simulink model "energy_storage_dclink"  (R2018a)
settings: Solver=ode4  StartTime=0.0  StopTime=sim.tTotal  FixedStep=sim.tStep  RelTol=1e-3
undefined symbols (not defined in the file or in its folder): D11, Delta, grid, sim, Vbase, vsc
libraries: powerlib x12, pwrsys x12
settings Model: Creator=ericfa  LastModifiedBy=ericfa

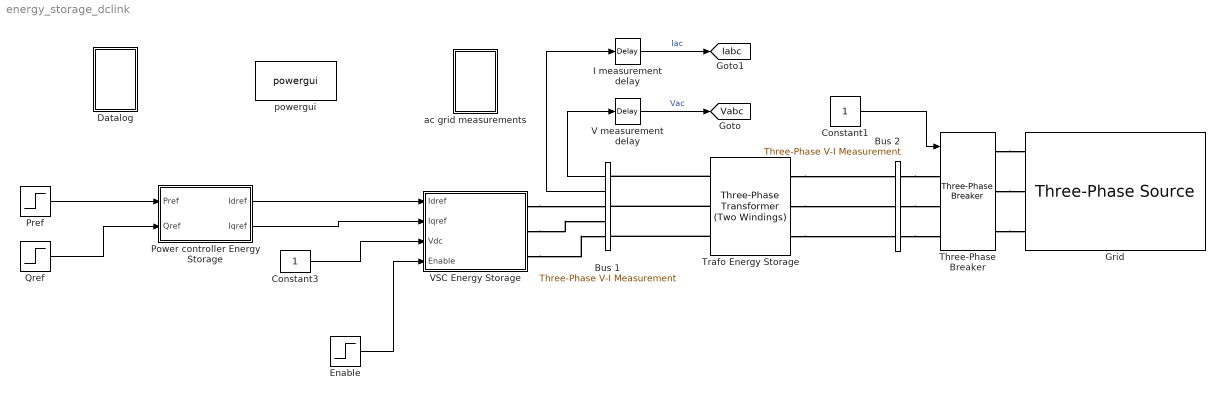
== system energy_storage_dclink ==
  Bus 1 : powerlib/Measurements/Three-Phase V-I Measurement  VoltageMeasurement=phase-to-ground  SetLabelV=off  LabelV=Vabc  Vpu=off  VpuLL=off  CurrentMeasurement=yes  SetLabelI=off  LabelI=Iabc  Ipu=off  Pbase=Sbase  Vbase=Vbase*sqrt(3/2)  OutputType=Complex  PhasorSimulation=off  PSBequivalent=0
  Bus 2 : powerlib/Measurements/Three-Phase V-I Measurement  VoltageMeasurement=phase-to-ground  SetLabelV=on  LabelV=Vabc_B2  Vpu=off  VpuLL=off  CurrentMeasurement=yes  SetLabelI=on  LabelI=Iabc_B2  Ipu=off  Pbase=100e6  Vbase=500e3  OutputType=Magnitude  PhasorSimulation=off  PSBequivalent=0
      settings: SourceProductName=Simscape Electrical
  Constant1 : Constant
  Constant3 : Constant
  Datalog : Subsystem
  Enable : Step  Time=0.05  SampleTime=0
  Grid : powerlib/Electrical Sources/Three-Phase Source  InternalConnection=Yg  VoltagePhases=off  Voltage=grid.UB2  PhaseAngle=0  Voltage_phases=[25e3 25e3 25e3]/sqrt(3)  PhaseAngles_phases=[0 -120 +120]  Frequency=grid.fn  NonIdealSource=on  SpecifyImpedance=on  Resistance=0.8929  Inductance=16.58e-3  ShortCircuitLevel=10*vsc.Sbase  BaseVoltage=grid.UB2  XRratio=10  BusType=swing  Pref=0  Qref=0  Prefabc=[10e3, 10e3, 10e3]  Qrefabc=[0, 0, 0]  Qmin=-inf  Qmax=inf
      settings: SourceProductName=Simscape Electrical
  I measurement delay : TransportDelay  DelayTime=sim.tStep; % 1/vsc.fSwitch
  Power controller Energy Storage : Subsystem
  Pref : Step  Time=0.4  After=0.5  SampleTime=0
  Qref : Step  Time=0.7  After=0.5  SampleTime=0
  Three-Phase Breaker : powerlib/Elements/Three-Phase Breaker  InitialState=open  SwitchA=on  SwitchB=on  SwitchC=on  SwitchTimes="[1/60  5/60]"  External=on  BreakerResistance=0.01  SnubberResistance=1e6  SnubberCapacitance=inf  Measurements=None
  Trafo Energy Storage : powerlib/Elements/Three-Phase Transformer (Two Windings)  Winding1Connection=Yg  Winding2Connection=Delta (D11)  CoreType=Three single-phase transformers  SetSaturation=off  Hysteresis=off  DataFile='hysteresis'  SetInitialFlux=off  Measurements=None  UNITS=pu  NominalPower=[ vsc.Sbase , grid.fn ]  Winding1=[ grid.UB1 , 0.002 , vsc.filterpu.Lg/2 ]  Winding2=[ grid.UB2 , 0.002 , vsc.filterpu.Lg/2 ]  Rm=200  Lm=200  L0=0.5  Saturation=[ 0,0 ; 0.0024,1.2 ; 1.0,1.52 ]  InitialFluxes=[ 0.8 , -0.8 , 0.7 ]  MoreParameters=off  BreakLoop=off  DataType=off  TransfoNumber=1
  V measurement delay : TransportDelay  DelayTime=sim.tStep; % 1/vsc.fSwitch
  VSC Energy Storage : Subsystem
  ac grid measurements : Subsystem
  powergui : powerlib/powergui  Priority=1  SimulationMode=Discrete  SampleTime=sim.tStep  frequency=60  Iterations=50  frequencyindice=60  Pbase=100e6  ErrMax=1e-4  UnitsV=kV  UnitsW=MW  buscounter=0  FunctionMessages=off  echomessages=off  EnableUseOfTLC=off  CurrentSourceSwitches=off  DisableSnubberDevices=off  DisableRonSwitches=off  DisableVfSwitches=off  DisplayEquations=off  SolverType=Tustin/Backward Euler (TBE)  Interpol=off  ExternalGateDelay=off  methode=off  Ts=100  x0status=steady  SPID=on  SwTol=0  HookPort=off  RestoreLinks=warning  ResistiveCurrentMeasurement=off  Frange=[0:2:500]  Ylog=off  Xlog=on  ShowGrid=off  save=off  variable=ZData  structure=0  ZoomFFT=off  StartTime=0.0  cycles=1  DisplayStyle=1  fundamental=60  FreqAxis=off  MaxFrequency=1000  frequencyindicesteady=1  RmsSteady=1  display=off
  tag scope: Iabc=global, Vabc=global
  wires:
  Constant1/1 -> Three-Phase Breaker/1
  Qref/1 -> Power controller Energy Storage/2(Qref)
  Enable/1 -> VSC Energy Storage/4(Enable)
  Pref/1 -> Power controller Energy Storage/1(Pref)
  Power controller Energy Storage/1(Idref) -> VSC Energy Storage/1(Idref)
  Power controller Energy Storage/2(Iqref) -> VSC Energy Storage/2(Iqref)
  V measurement delay/1 -> [Vabc]  "Vac"
  Bus 1/2 -> I measurement delay/1
  Bus 1/1 -> V measurement delay/1
  I measurement delay/1 -> [Iabc]  "Iac"
  Constant3/1 -> VSC Energy Storage/3(Vdc)
  connections:
  Bus 2/RConn1 -- Three-Phase Breaker/LConn1
  Bus 2/RConn2 -- Three-Phase Breaker/LConn2
  Bus 2/RConn3 -- Three-Phase Breaker/LConn3
  Three-Phase Breaker/RConn1 -- Grid/RConn1
  Three-Phase Breaker/RConn2 -- Grid/RConn2
  Three-Phase Breaker/RConn3 -- Grid/RConn3
  Trafo Energy Storage/RConn1 -- Bus 2/LConn1
  VSC Energy Storage/RConn1 -- Bus 1/RConn1
  VSC Energy Storage/RConn2 -- Bus 1/RConn2
  VSC Energy Storage/RConn3 -- Bus 1/RConn3
  Trafo Energy Storage/RConn2 -- Bus 2/LConn2
  Trafo Energy Storage/RConn3 -- Bus 2/LConn3
  Trafo Energy Storage/LConn3 -- Bus 1/LConn3
  Trafo Energy Storage/LConn2 -- Bus 1/LConn2
  Trafo Energy Storage/LConn1 -- Bus 1/LConn1

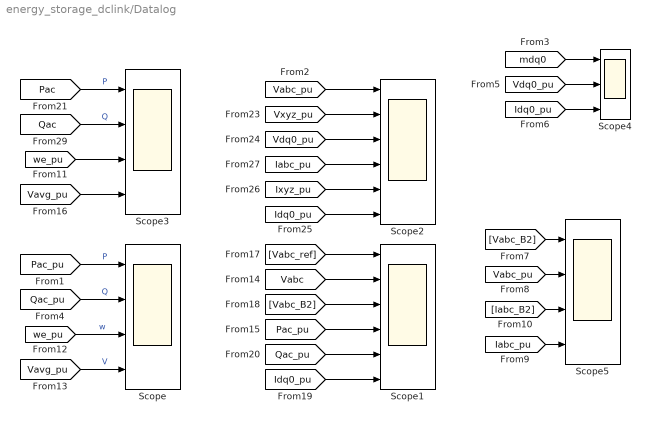
== system energy_storage_dclink/Datalog ==
  Scope : Scope  NumInputPorts=4
  Scope1 : Scope  NumInputPorts=6
  Scope2 : Scope  NumInputPorts=6
  Scope3 : Scope  NumInputPorts=4
  Scope4 : Scope  NumInputPorts=3
  Scope5 : Scope  NumInputPorts=4
  wires:
  [Qac_pu] -> Scope1/5
  [Vavg_pu] -> Scope/4  "V"
  [Idq0_pu] -> Scope2/6
  [Idq0_pu] -> Scope1/6
  [Vabc] -> Scope1/2
  [we_pu] -> Scope/3  "w"
  [Vxyz_pu] -> Scope2/2
  [Qac_pu] -> Scope/2  "Q"
  [Pac] -> Scope3/1  "P"
  [Vabc_ref] -> Scope1/1
  [Vabc_pu] -> Scope2/1
  [Vabc_B2] -> Scope1/3
  [Pac_pu] -> Scope1/4
  [Iabc_pu] -> Scope2/4
  [Ixyz_pu] -> Scope2/5
  [Qac] -> Scope3/2  "Q"
  [Pac_pu] -> Scope/1  "P"
  [Vdq0_pu] -> Scope2/3
  [Vdq0_pu] -> Scope4/2
  [mdq0] -> Scope4/1
  [Idq0_pu] -> Scope4/3
  [Vabc_B2] -> Scope5/1
  [Vabc_pu] -> Scope5/2
  [Iabc_pu] -> Scope5/4
  [Iabc_B2] -> Scope5/3
  [we_pu] -> Scope3/3
  [Vavg_pu] -> Scope3/4

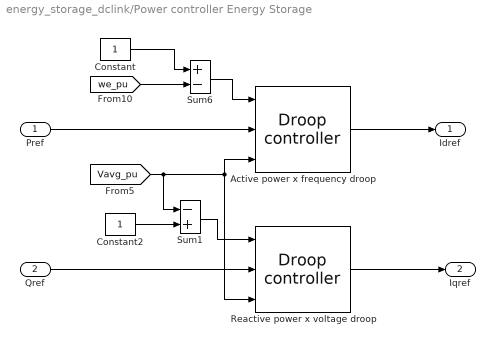
== system energy_storage_dclink/Power controller Energy Storage ==
  Pref : Inport
  Qref : Inport  Port=2
  Active power x frequency droop : pwrsys/Controllers/Droop controller  Refmax=1  Refmin=-1  Kp=vsc.Pdroop.Kp  Kd=vsc.Pdroop.Kd  Tr=vsc.Pdroop.Tr  flp=vsc.Pdroop.flp  DB=vsc.Pdroop.DB
      settings: SourceProductName=NTNU Power Systems
  Constant : Constant
  Constant2 : Constant
  Reactive power x voltage droop : pwrsys/Controllers/Droop controller  Refmax=1  Refmin=-1  Kp=vsc.Qdroop.Kp  Kd=vsc.Qdroop.Kd  Tr=vsc.Qdroop.Tr  flp=vsc.Qdroop.flp  DB=vsc.Qdroop.DB
      settings: SourceProductName=NTNU Power Systems
  Sum1 : Sum  Inputs=-+
  Sum6 : Sum  Inputs=+-
  Idref : Outport
  Iqref : Outport  Port=2
  wires:
  [Vavg_pu] -> Reactive power x voltage droop/3, Active power x frequency droop/3, Sum1/1
  Constant/1 -> Sum6/1
  Qref/1 -> Reactive power x voltage droop/2
  Reactive power x voltage droop/1 -> Iqref/1
  [we_pu] -> Sum6/2
  Pref/1 -> Active power x frequency droop/2
  Sum1/1 -> Reactive power x voltage droop/1
  Sum6/1 -> Active power x frequency droop/1
  Constant2/1 -> Sum1/2
  Active power x frequency droop/1 -> Idref/1

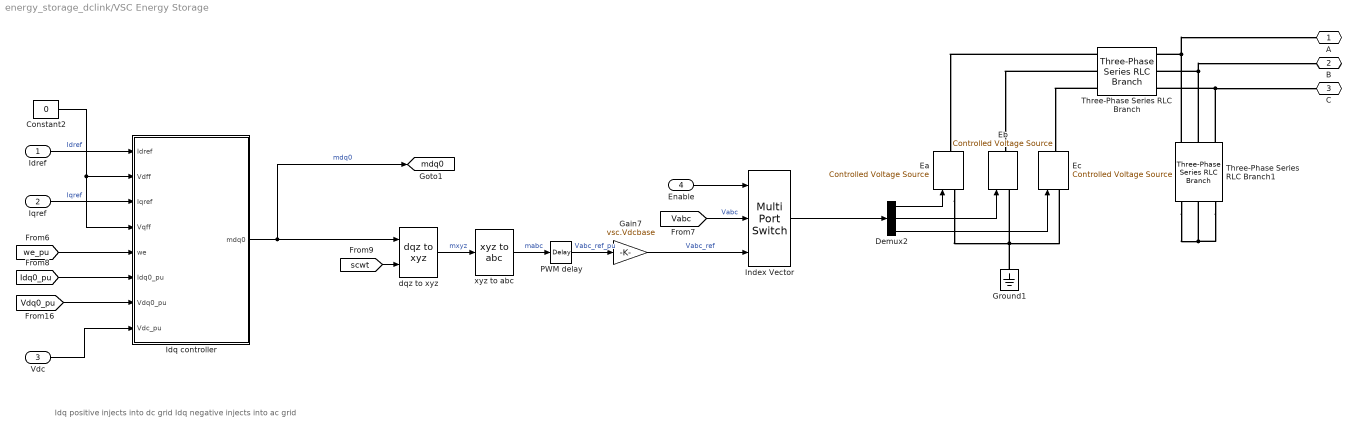
== system energy_storage_dclink/VSC Energy Storage ==
  note: Idq positive injects into dc grid
      | Idq negative injects into ac grid
  Idref : Inport
  Iqref : Inport  Port=2
  Vdc : Inport  Port=3
  Enable : Inport  Port=4
  Constant2 : Constant  Value=0
  Demux2 : Demux  Outputs=3
  Ea : powerlib/Electrical Sources/Controlled Voltage Source  Initialize=on  Source_Type=AC  Amplitude=vsc.Vbase  Phase=0  Frequency=vsc.fbase  Measurements=None
  Eb : powerlib/Electrical Sources/Controlled Voltage Source  Initialize=on  Source_Type=AC  Amplitude=vsc.Vbase  Phase=-120  Frequency=vsc.fbase  Measurements=None
  Ec : powerlib/Electrical Sources/Controlled Voltage Source  Initialize=on  Source_Type=AC  Amplitude=vsc.Vbase  Phase=120  Frequency=vsc.fbase  Measurements=None
  Gain7 : Gain  Gain=vsc.Vdcbase
  Ground1 : powerlib/Elements/Ground  LConnTagsString=a
  Idq controller : Subsystem  mask{Imax=1, mmax=vsc.mmax, K=vsc.ctrl.kvsc, Lf=vsc.filterpu.Lac, Rf=vsc.filterpu.Rac, fLC=vsc.ctrl.ffilt, Ts=1/vsc.fSwitch, kp=vsc.ctrl.kp, ki=vsc.ctrl.ki, Kff=1}
      mask prompts: Imax "Maximum AC current"; mmax "Maximum modulation index (PWM gain)"; K "Converter gain (Vdcbase/Vbase)"; Lf "AC filter - L value"; Rf "AC filter - R value"; fLC "AC filter cut-off frequency"; Ts "Sampling time"; Kff "Kff (1 = enable voltage feed-forward)"
      mask DialogControl Container4 Prompt: Controller gains
  Index Vector : MultiPortSwitch  DataPortOrder=Zero-based contiguous  Inputs=2  zeroidx=on
  PWM delay : TransportDelay  DelayTime=sim.tStep; % 1/vsc.fSwitch
  Three-Phase Series RLC Branch : powerlib/Elements/Three-Phase Series RLC Branch  LConnTagsString=A|B|C  RConnTagsString=A|B|C  BranchType=RL  Resistance=vsc.filter.Rac  Inductance=vsc.filter.Lac  Capacitance=1e-6  Measurements=None
  Three-Phase Series RLC Branch1 : powerlib/Elements/Three-Phase Series RLC Branch  LConnTagsString=A|B|C  RConnTagsString=A|B|C  BranchType=RC  Resistance=vsc.filter.Rlc  Inductance=vsc.filter.Lac  Capacitance=vsc.filter.Clc  Measurements=None
  dqz to xyz : pwrsys/Transformations/dqz to xyz  SystemSampleTime=-1
      settings: SourceProductName=NTNU Power Systems
  xyz to abc : pwrsys/Transformations/xyz to abc  typeTransf=Amplitude-invariant
      settings: SourceProductName=NTNU Power Systems
  A : PMIOPort  Side=Right
  B : PMIOPort  Port=2  Side=Right
  C : PMIOPort  Port=3  Side=Right
  tag scope: mdq0=global
  wires:
  Demux2/2 -> Eb/1
  Demux2/1 -> Ea/1
  Demux2/3 -> Ec/1
  Index Vector/1 -> Demux2/1
  Idq controller/1(mdq0) -> [mdq0], dqz to xyz/1  "mdq0"
  [Idq0_pu] -> Idq controller/6(Idq0_pu)
  [we_pu] -> Idq controller/5(we)
  [Vdq0_pu] -> Idq controller/7(Vdq0_pu)
  [Vabc] -> Index Vector/2  "Vabc"
  [scwt] -> dqz to xyz/2
  xyz to abc/1 -> PWM delay/1  "mabc"
  PWM delay/1 -> Gain7/1  "Vabc_ref_pu"
  Gain7/1 -> Index Vector/3  "Vabc_ref"
  Constant2/1 -> Idq controller/4(Vqff), Idq controller/2(Vdff)
  Vdc/1 -> Idq controller/8(Vdc_pu)
  dqz to xyz/1 -> xyz to abc/1  "mxyz"
  Enable/1 -> Index Vector/1
  Idref/1 -> Idq controller/1(Idref)  "Idref"
  Iqref/1 -> Idq controller/3(Iqref)  "Iqref"
  connections:
  Three-Phase Series RLC Branch/RConn1 -- Ea/RConn1
  Three-Phase Series RLC Branch/RConn2 -- Eb/RConn1
  Three-Phase Series RLC Branch/RConn3 -- Ec/RConn1
  Three-Phase Series RLC Branch/LConn1 -- A/RConn1 -- Three-Phase Series RLC Branch1/LConn1
  Three-Phase Series RLC Branch/LConn2 -- B/RConn1 -- Three-Phase Series RLC Branch1/LConn2
  Three-Phase Series RLC Branch/LConn3 -- C/RConn1 -- Three-Phase Series RLC Branch1/LConn3
  Ea/LConn1 -- Eb/LConn1 -- Ground1/LConn1 -- Ec/LConn1
  Three-Phase Series RLC Branch1/RConn3 -- Three-Phase Series RLC Branch1/RConn2 -- Three-Phase Series RLC Branch1/RConn1

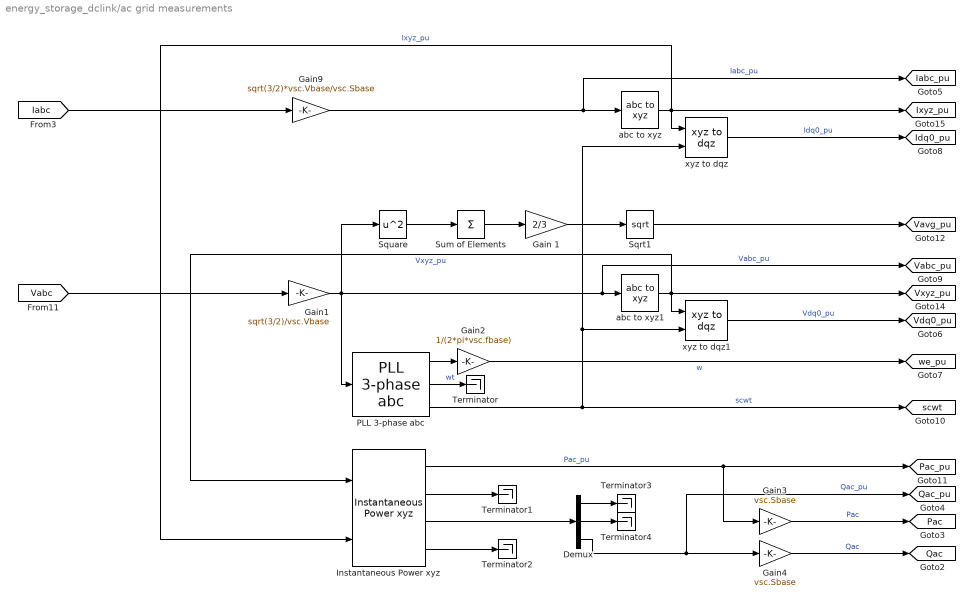
== system energy_storage_dclink/ac grid measurements ==
  Demux : Demux  Outputs=3
  "Gain 1 " : Gain  Gain=2/3
  Gain1 : Gain  Gain=sqrt(3/2)/vsc.Vbase
  Gain2 : Gain  Gain=1/(2*pi*vsc.fbase)
  Gain3 : Gain  Gain=vsc.Sbase
  Gain4 : Gain  Gain=vsc.Sbase
  Gain9 : Gain  Gain=sqrt(3/2)*vsc.Vbase/vsc.Sbase
  Instantaneous Power xyz : pwrsys/Measurement/Instantaneous Power xyz  typeTransf=Amplitude-invariant
      settings: SourceProductName=NTNU Power Systems
  PLL 3-phase abc : pwrsys/PLLs/PLL 3-phase abc  fnom=vsc.fbase  fdev=1/3*vsc.fbase  zeta=0.707  Kp=vsc.pll.Kp  Ki=vsc.pll.Ki  Kd=vsc.pll.Kd  Tr=vsc.pll.Tr  Ts=vsc.fSwitch
      settings: SourceProductName=NTNU Power Systems
  Sqrt1 : Sqrt  SaturateOnIntegerOverflow=on
  Square : Math  Operator=square  SaturateOnIntegerOverflow=on
  Sum of Elements : Sum  Inputs=+
  Terminator{,1..4} (5 alike) : Terminator
  abc to xyz : pwrsys/Transformations/abc to xyz  typeTransf=Amplitude-invariant
      settings: SourceProductName=NTNU Power Systems
  abc to xyz1 : pwrsys/Transformations/abc to xyz  typeTransf=Amplitude-invariant
      settings: SourceProductName=NTNU Power Systems
  xyz to dqz : pwrsys/Transformations/xyz to dqz  SystemSampleTime=-1
      settings: SourceProductName=NTNU Power Systems
  xyz to dqz1 : pwrsys/Transformations/xyz to dqz  SystemSampleTime=-1
      settings: SourceProductName=NTNU Power Systems
  tag scope: Iabc_pu=global, Idq0_pu=global, Ixyz_pu=global, Pac=global, Pac_pu=global, Qac=global, Qac_pu=global, Vabc_pu=global, Vavg_pu=global, Vdq0_pu=global, Vxyz_pu=global, scwt=global, we_pu=global
  wires:
  Sqrt1/1 -> [Vavg_pu]
  Gain4/1 -> [Qac]  "Qac"
  Gain3/1 -> [Pac]  "Pac"
  Demux/2 -> Terminator4/1
  Demux/1 -> Terminator3/1
  Instantaneous Power xyz/3 -> Demux/1
  Instantaneous Power xyz/4 -> Terminator2/1
  Instantaneous Power xyz/2 -> Terminator1/1
  PLL 3-phase abc/2 -> Terminator/1  "wt"
  abc to xyz1/1 -> [Vxyz_pu], xyz to dqz1/1, Instantaneous Power xyz/1  "Vxyz_pu"
  abc to xyz/1 -> [Ixyz_pu], xyz to dqz/1, Instantaneous Power xyz/2  "Ixyz_pu"
  "Gain 1 "/1 -> Sqrt1/1
  Sum of Elements/1 -> "Gain 1 "/1
  Square/1 -> Sum of Elements/1
  Demux/3 -> [Qac_pu], Gain4/1  "Qac_pu"
  Instantaneous Power xyz/1 -> Gain3/1, [Pac_pu]  "Pac_pu"
  [Vabc] -> Gain1/1
  [Iabc] -> Gain9/1
  xyz to dqz1/1 -> [Vdq0_pu]  "Vdq0_pu"
  PLL 3-phase abc/1 -> Gain2/1
  Gain2/1 -> [we_pu]  "w"
  PLL 3-phase abc/3 -> [scwt], xyz to dqz/2, xyz to dqz1/2  "scwt"
  Gain1/1 -> Square/1, PLL 3-phase abc/1, [Vabc_pu], abc to xyz1/1  "Vabc_pu"
  xyz to dqz/1 -> [Idq0_pu]  "Idq0_pu"
  Gain9/1 -> [Iabc_pu], abc to xyz/1  "Iabc_pu"

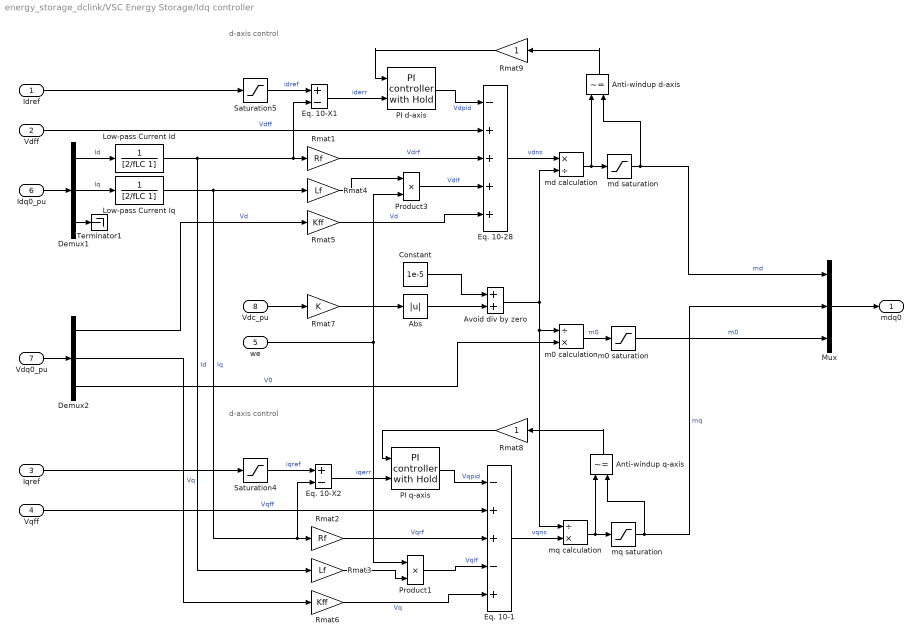
== system energy_storage_dclink/VSC Energy Storage/Idq controller ==
  note: d-axis control
  note: d-axis control
  Idref : Inport
  Vdff : Inport  Port=2
  Iqref : Inport  Port=3
  Vqff : Inport  Port=4
  we : Inport  Port=5
  Idq0_pu : Inport  Port=6
  Vdq0_pu : Inport  Port=7
  Vdc_pu : Inport  Port=8
  Abs : Abs  ZeroCross=off
  Anti-windup d-axis : RelationalOperator  Operator=~=  OutDataTypeStr=boolean  RndMeth=Simplest
  Anti-windup q-axis : RelationalOperator  Operator=~=  OutDataTypeStr=boolean  RndMeth=Simplest
  Avoid div by zero : Sum
  Constant : Constant  Value=1e-5
  Demux1 : Demux  Outputs=3
  Demux2 : Demux  Outputs=3
  Eq. 10-1 : Sum  Inputs=-++-+  SaturateOnIntegerOverflow=on  InputSameDT=on  OutDataTypeStr=Inherit: Same as first input
  Eq. 10-28 : Sum  Inputs=-++++  SaturateOnIntegerOverflow=on  InputSameDT=on  OutDataTypeStr=Inherit: Same as first input
  Eq. 10-X1 : Sum  Inputs=+-  SaturateOnIntegerOverflow=on  InputSameDT=on  OutDataTypeStr=Inherit: Same as first input
  Eq. 10-X2 : Sum  Inputs=+-  SaturateOnIntegerOverflow=on  InputSameDT=on  OutDataTypeStr=Inherit: Same as first input
  Low-pass Current Id : TransferFcn  Denominator=[2/fLC 1]
  Low-pass Current Iq : TransferFcn  Denominator=[2/fLC 1]
  Mux : Mux  Inputs=3
  PI d-axis : pwrsys/Controllers/PI controller  with Hold  Kp=kp  Ki=ki  Max=K*mmax  Min=-K*mmax  x0=0  Ts=Ts
      settings: SourceProductName=NTNU Power Systems
  PI q-axis : pwrsys/Controllers/PI controller  with Hold  Kp=kp  Ki=ki  Max=K*mmax  Min=-K*mmax  x0=0  Ts=Ts
      settings: SourceProductName=NTNU Power Systems
  Product1 : Product  SaturateOnIntegerOverflow=on  RndMeth=Zero  InputSameDT=on  OutDataTypeStr=Inherit: Same as first input
  Product3 : Product  SaturateOnIntegerOverflow=on  RndMeth=Zero  InputSameDT=on  OutDataTypeStr=Inherit: Same as first input
  Rmat1 : Gain  Gain=Rf
  Rmat2 : Gain  Gain=Rf
  Rmat3 : Gain  Gain=Lf
  Rmat4 : Gain  Gain=Lf
  Rmat5 : Gain  Gain=Kff
  Rmat6 : Gain  Gain=Kff
  Rmat7 : Gain  Gain=K
  Rmat8 : Gain
  Rmat9 : Gain
  Saturation4 : Saturate  UpperLimit=Imax  LowerLimit=-Imax
  Saturation5 : Saturate  UpperLimit=Imax  LowerLimit=-Imax
  Terminator1 : Terminator
  m0 saturation : Saturate  UpperLimit=mmax  LowerLimit=-mmax
  m0 calculation : Product  Inputs=/*
  md calculation : Product  Inputs=*/
  md saturation : Saturate  UpperLimit=mmax  LowerLimit=-mmax
  mq saturation : Saturate  UpperLimit=mmax  LowerLimit=-mmax
  mq calculation : Product  Inputs=/*
  mdq0 : Outport
  wires:
  Idref/1 -> Saturation5/1
  Iqref/1 -> Saturation4/1
  Demux1/3 -> Terminator1/1
  Vdq0_pu/1 -> Demux2/1
  Mux/1 -> mdq0/1
  Demux2/3 -> m0 calculation/2  "V0"
  Product3/1 -> Eq. 10-28/4  "Vdlf"
  Rmat4/1 -> Product3/1
  md saturation/1 -> Anti-windup d-axis/2, Mux/1  "md"
  Anti-windup d-axis/1 -> Rmat9/1
  PI d-axis/1 -> Eq. 10-28/1  "Vdpid"
  Eq. 10-28/1 -> md calculation/1  "vdns"
  Saturation5/1 -> Eq. 10-X1/1  "idref"
  Demux2/1 -> Rmat5/1  "Vd"
  Rmat5/1 -> Eq. 10-28/5  "Vd"
  Vdff/1 -> Eq. 10-28/2  "Vdff"
  Demux1/2 -> Low-pass Current Iq/1  "Iq"
  Rmat6/1 -> Eq. 10-1/5  "Vq"
  Saturation4/1 -> Eq. 10-X2/1  "iqref"
  mq saturation/1 -> Mux/2, Anti-windup q-axis/2  "mq"
  Rmat3/1 -> Product1/2
  Anti-windup q-axis/1 -> Rmat8/1
  Demux1/1 -> Low-pass Current Id/1  "Id"
  Vqff/1 -> Eq. 10-1/2  "Vqff"
  Eq. 10-1/1 -> mq calculation/2  "vqns"
  Demux2/2 -> Rmat6/1  "Vq"
  Product1/1 -> Eq. 10-1/4  "Vqlf"
  Eq. 10-X2/1 -> PI q-axis/2  "iqerr"
  we/1 -> Product3/2, Product1/1
  PI q-axis/1 -> Eq. 10-1/1  "Vqpid"
  Idq0_pu/1 -> Demux1/1
  Low-pass Current Id/1 -> Eq. 10-X1/2, Rmat1/1, Rmat3/1  "Id"
  Low-pass Current Iq/1 -> Eq. 10-X2/2, Rmat2/1, Rmat4/1  "Iq"
  Rmat2/1 -> Eq. 10-1/3  "Vqrf"
  Rmat1/1 -> Eq. 10-28/3  "Vdrf"
  Eq. 10-X1/1 -> PI d-axis/2  "iderr"
  Avoid div by zero/1 -> m0 calculation/1, mq calculation/1, md calculation/2
  Constant/1 -> Avoid div by zero/1
  Abs/1 -> Avoid div by zero/2
  md calculation/1 -> Anti-windup d-axis/1, md saturation/1
  mq calculation/1 -> mq saturation/1, Anti-windup q-axis/1
  m0 calculation/1 -> m0 saturation/1  "m0"
  Vdc_pu/1 -> Rmat7/1
  Rmat7/1 -> Abs/1
  m0 saturation/1 -> Mux/3  "m0"
  Rmat8/1 -> PI q-axis/1
  Rmat9/1 -> PI d-axis/1
